simulink library "config"  (R2024b)
settings: Solver=VariableStepAuto  StartTime=0.0  StopTime=10.0  RelTol=1e-3
settings Model: Creator=mainuser  LastModifiedBy=mainuser

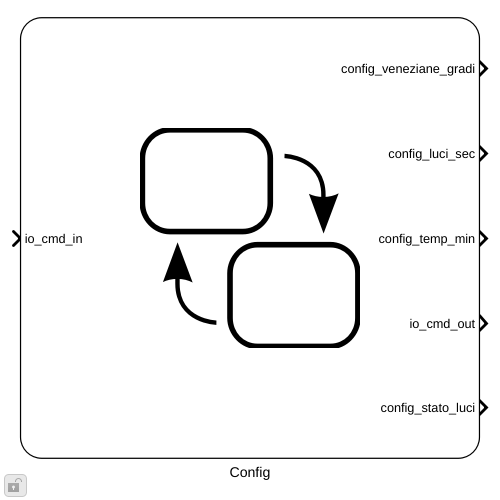
[thumbnail: Simulink's stored preview of the top-level diagram]
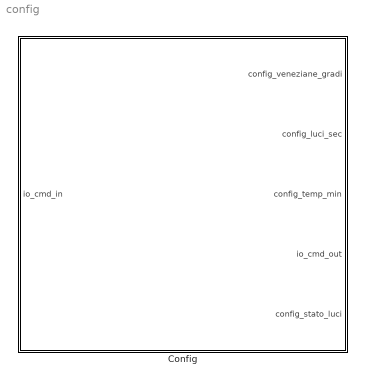
== system config ==
  Config : Stateflow chart  TreatAsAtomicUnit=on

== stateflow chart config/Config ==
  state AA
    config_stato_luci=0
    io_cmd_out=""
    config_luci_sec=0
    config_temp_min=0
    config_veneziane_gradi=0
  (default) -> AA
  AA -> 114
  data: veneziane_gradi function_input double size=1; temperatura_gradi function_input double size=1; luci_secondi function_input double size=1; err function_output string; err function_output string; gradi function_input double size=1; temp function_input double size=1; err function_output string; sec function_input double size=1; err function_output string; io_cmd_in input int8; config_veneziane_gradi output; config_luci_sec output; config_temp_min output; io_cmd_out output string; change_veneziane_gradi local =0; change_luci_sec local =0; change_temp_min local =0; config_stato_luci output
  function err = checkAll(veneziane_gradi,temperatura_gradi,luci_secondi):
    | function err = checkAll(veneziane_gradi,temperatura_gradi,luci_secondi)
    | 
    | err = checkVeneziane(veneziane_gradi)
    | if err~=""
    |     return
    | end
    | 
    | err = checkTemperatura(temperatura_gradi)
    | if err~=""
    |     return
    | end
    | 
    | err = checkLuciSec(luci_secondi)
    | if err~=""
    |     return
    | end
    | 
    | end
  function err = checkVeneziane(gradi):
    | function err = checkVeneziane(gradi)
    |  if gradi<0
    |      err="Numero gradi negativo";
    |  elseif gradi>180
    |      err="Numero gradi troppo grande (al massimo 180 gradi)";
    |  elseif ~mod(gradi,20)
    |     err="Numero gradi troppo precisio (passo supportato 20 gradi)"
    |  else
    |      err="";
    |  end
    | end
  function err = checkTemperatura(temp):
    | function err = checkTemperatura(temp)
    |     if temp<16
    |         err="temperatura troppo bassa (almeno 16)";
    |     elseif temp>30
    |         err="temperatura troppo alta (al massimo 30)";
    |     elseif ~mod(temp,1)
    |         err="temperatura troppo precisia (passo supportato 1 grado)"
    |     else
    |        err="";
    |     end
    | end
  function err = checkLuciSec(sec):
    | function err = checkLuciSec(sec)
    |     if sec==0
    |         err=""
    |     elseif sec<5
    |         err="troppi pochi secondi (almeno 5)";
    |     elseif sec>30
    |         err="troppi secondi (al massimo 30)";
    |     elseif ~mod(sec,1)
    |         err="numero secondi troppo precisio (passo supportato 1 secondo)"
    |     else
    |        err="";
    |     end
    | end
